simulink model "VCU_CS75_9_30"  (R2014a)
settings: Solver=FixedStepDiscrete  StartTime=0.0  StopTime=25  FixedStep=0.0005  RelTol=1e-3
undefined symbols (not defined in the file or in its folder): APAStatus_2D4, ecucoder_acal, I_SW01_L, LDW, ST_comd, TX2D4
libraries: simulink x881, ec5744lib x37
(part 8 of 30)

== system VCU_CS75_9_30/长安CS75底盘程序，20ms一次/BSW_Input/DBC转化的messages（存底）/ReceiveMessages4/EPB_256 ==
  input : Inport
  Demux : Demux  Outputs=8
  EPB_Checksum_Ad : Sum
  EPB_Checksum_Convert : DataTypeConversion  OutDataTypeStr=uint32
  EPB_Checksum_F : Gain
  EPB_Checksum_L : simulink/Logic and Bit Operations/Bitwise Operator  logicop=AND  UseBitMask=on  BitMask=255  BitMaskRealWorld=Stored Integer
  EPB_Checksum_O : Constant  Value=0  OutDataTypeStr=single
  EPB_Checksum_S : ArithShift
  EPB_Checksum_Sub : Subsystem
  EPB_Checksum_sat : Saturate  UpperLimit=255  LowerLimit=0
  EPB_Checksumcv : DataTypeConversion
  EPB_FailStatus_Ad : Sum
  EPB_FailStatus_Convert : DataTypeConversion  OutDataTypeStr=uint32
  EPB_FailStatus_F : Gain
  EPB_FailStatus_L : simulink/Logic and Bit Operations/Bitwise Operator  logicop=AND  UseBitMask=on  BitMask=192  BitMaskRealWorld=Stored Integer
  EPB_FailStatus_O : Constant  Value=0  OutDataTypeStr=single
  EPB_FailStatus_S : ArithShift  BitShiftNumber=6
  EPB_FailStatus_Sub : Subsystem
  EPB_FailStatus_sat : Saturate  UpperLimit=3  LowerLimit=0
  EPB_FailStatuscv : DataTypeConversion
  EPB_FailureLamp_Ad : Sum
  EPB_FailureLamp_Convert : DataTypeConversion  OutDataTypeStr=uint32
  EPB_FailureLamp_F : Gain
  EPB_FailureLamp_L : simulink/Logic and Bit Operations/Bitwise Operator  logicop=AND  UseBitMask=on  BitMask=48  BitMaskRealWorld=Stored Integer
  EPB_FailureLamp_O : Constant  Value=0  OutDataTypeStr=single
  EPB_FailureLamp_S : ArithShift  BitShiftNumber=4
  EPB_FailureLamp_Sub : Subsystem
  EPB_FailureLamp_sat : Saturate  UpperLimit=3  LowerLimit=0
  EPB_FailureLampcv : DataTypeConversion
  EPB_FunctionLamp_Ad : Sum
  EPB_FunctionLamp_Convert : DataTypeConversion  OutDataTypeStr=uint32
  EPB_FunctionLamp_F : Gain
  EPB_FunctionLamp_L : simulink/Logic and Bit Operations/Bitwise Operator  logicop=AND  UseBitMask=on  BitMask=12  BitMaskRealWorld=Stored Integer
  EPB_FunctionLamp_O : Constant  Value=0  OutDataTypeStr=single
  EPB_FunctionLamp_S : ArithShift  BitShiftNumber=2
  EPB_FunctionLamp_Sub : Subsystem
  EPB_FunctionLamp_sat : Saturate  UpperLimit=3  LowerLimit=0
  EPB_FunctionLampcv : DataTypeConversion
  EPB_RollingCounter_id256_Ad : Sum
  EPB_RollingCounter_id256_Convert : DataTypeConversion  OutDataTypeStr=uint32
  EPB_RollingCounter_id256_F : Gain
  EPB_RollingCounter_id256_L : simulink/Logic and Bit Operations/Bitwise Operator  logicop=AND  UseBitMask=on  BitMask=15  BitMaskRealWorld=Stored Integer
  EPB_RollingCounter_id256_O : Constant  Value=0  OutDataTypeStr=single
  EPB_RollingCounter_id256_S : ArithShift
  EPB_RollingCounter_id256_Sub : Subsystem
  EPB_RollingCounter_id256_sat : Saturate  UpperLimit=15  LowerLimit=0
  EPB_RollingCounter_id256cv : DataTypeConversion
  EPB_Status_Ad : Sum
  EPB_Status_Convert : DataTypeConversion  OutDataTypeStr=uint32
  EPB_Status_F : Gain
  EPB_Status_L : simulink/Logic and Bit Operations/Bitwise Operator  logicop=AND  UseBitMask=on  BitMask=192  BitMaskRealWorld=Stored Integer
  EPB_Status_O : Constant  Value=0  OutDataTypeStr=single
  EPB_Status_S : ArithShift  BitShiftNumber=6
  EPB_Status_Sub : Subsystem
  EPB_Status_sat : Saturate  UpperLimit=3  LowerLimit=0
  EPB_Statuscv : DataTypeConversion
  EPB_FailStatus_Out : Outport
  EPB_Status_Out : Outport  Port=2
  EPB_FunctionLamp_Out : Outport  Port=3
  EPB_FailureLamp_Out : Outport  Port=4
  EPB_RollingCounter_id256_Out : Outport  Port=5
  EPB_Checksum_Out : Outport  Port=6
  wires:
  EPB_FailStatus_F/1 -> EPB_FailStatus_Ad/1
  EPB_FailStatus_O/1 -> EPB_FailStatus_Ad/2
  EPB_FailStatus_Ad/1 -> EPB_FailStatus_sat/1
  EPB_FailStatus_sat/1 -> EPB_FailStatus_Out/1
  Demux/1 -> EPB_FailStatus_Sub/1(In1)
  EPB_FailStatus_Sub/1(Out1) -> EPB_FailStatus_Convert/1
  EPB_FailStatus_Convert/1 -> EPB_FailStatus_L/1
  EPB_FailStatus_L/1 -> EPB_FailStatus_S/1
  EPB_FailStatus_S/1 -> EPB_FailStatuscv/1
  EPB_FailStatuscv/1 -> EPB_FailStatus_F/1
  EPB_Status_F/1 -> EPB_Status_Ad/1
  EPB_Status_O/1 -> EPB_Status_Ad/2
  EPB_Status_Ad/1 -> EPB_Status_sat/1
  EPB_Status_sat/1 -> EPB_Status_Out/1
  Demux/3 -> EPB_Status_Sub/1(In1)
  EPB_Status_Sub/1(Out1) -> EPB_Status_Convert/1
  EPB_Status_Convert/1 -> EPB_Status_L/1
  EPB_Status_L/1 -> EPB_Status_S/1
  EPB_Status_S/1 -> EPB_Statuscv/1
  EPB_Statuscv/1 -> EPB_Status_F/1
  EPB_FunctionLamp_F/1 -> EPB_FunctionLamp_Ad/1
  EPB_FunctionLamp_O/1 -> EPB_FunctionLamp_Ad/2
  EPB_FunctionLamp_Ad/1 -> EPB_FunctionLamp_sat/1
  EPB_FunctionLamp_sat/1 -> EPB_FunctionLamp_Out/1
  Demux/6 -> EPB_FunctionLamp_Sub/1(In1), EPB_FailureLamp_Sub/1(In1)
  EPB_FunctionLamp_Sub/1(Out1) -> EPB_FunctionLamp_Convert/1
  EPB_FunctionLamp_Convert/1 -> EPB_FunctionLamp_L/1
  EPB_FunctionLamp_L/1 -> EPB_FunctionLamp_S/1
  EPB_FunctionLamp_S/1 -> EPB_FunctionLampcv/1
  EPB_FunctionLampcv/1 -> EPB_FunctionLamp_F/1
  EPB_FailureLamp_F/1 -> EPB_FailureLamp_Ad/1
  EPB_FailureLamp_O/1 -> EPB_FailureLamp_Ad/2
  EPB_FailureLamp_Ad/1 -> EPB_FailureLamp_sat/1
  EPB_FailureLamp_sat/1 -> EPB_FailureLamp_Out/1
  EPB_FailureLamp_Sub/1(Out1) -> EPB_FailureLamp_Convert/1
  EPB_FailureLamp_Convert/1 -> EPB_FailureLamp_L/1
  EPB_FailureLamp_L/1 -> EPB_FailureLamp_S/1
  EPB_FailureLamp_S/1 -> EPB_FailureLampcv/1
  EPB_FailureLampcv/1 -> EPB_FailureLamp_F/1
  EPB_RollingCounter_id256_F/1 -> EPB_RollingCounter_id256_Ad/1
  EPB_RollingCounter_id256_O/1 -> EPB_RollingCounter_id256_Ad/2
  EPB_RollingCounter_id256_Ad/1 -> EPB_RollingCounter_id256_sat/1
  EPB_RollingCounter_id256_sat/1 -> EPB_RollingCounter_id256_Out/1
  Demux/7 -> EPB_RollingCounter_id256_Sub/1(In1)
  EPB_RollingCounter_id256_Sub/1(Out1) -> EPB_RollingCounter_id256_Convert/1
  EPB_RollingCounter_id256_Convert/1 -> EPB_RollingCounter_id256_L/1
  EPB_RollingCounter_id256_L/1 -> EPB_RollingCounter_id256_S/1
  EPB_RollingCounter_id256_S/1 -> EPB_RollingCounter_id256cv/1
  EPB_RollingCounter_id256cv/1 -> EPB_RollingCounter_id256_F/1
  EPB_Checksum_F/1 -> EPB_Checksum_Ad/1
  EPB_Checksum_O/1 -> EPB_Checksum_Ad/2
  EPB_Checksum_Ad/1 -> EPB_Checksum_sat/1
  EPB_Checksum_sat/1 -> EPB_Checksum_Out/1
  Demux/8 -> EPB_Checksum_Sub/1(In1)
  EPB_Checksum_Sub/1(Out1) -> EPB_Checksum_Convert/1
  EPB_Checksum_Convert/1 -> EPB_Checksum_L/1
  EPB_Checksum_L/1 -> EPB_Checksum_S/1
  EPB_Checksum_S/1 -> EPB_Checksumcv/1
  EPB_Checksumcv/1 -> EPB_Checksum_F/1
  input/1 -> Demux/1

== system VCU_CS75_9_30/长安CS75底盘程序，20ms一次/BSW_Input/DBC转化的messages（存底）/ReceiveMessages5/EPS_20A ==
  input : Inport
  Demux : Demux  Outputs=8
  EPS_APA_AbortFeedback_Ad : Sum
  EPS_APA_AbortFeedback_Convert : DataTypeConversion  OutDataTypeStr=uint32
  EPS_APA_AbortFeedback_F : Gain
  EPS_APA_AbortFeedback_L : simulink/Logic and Bit Operations/Bitwise Operator  logicop=AND  UseBitMask=on  BitMask=112  BitMaskRealWorld=Stored Integer
  EPS_APA_AbortFeedback_O : Constant  Value=0  OutDataTypeStr=single
  EPS_APA_AbortFeedback_S : ArithShift  BitShiftNumber=4
  EPS_APA_AbortFeedback_Sub : Subsystem
  EPS_APA_AbortFeedback_sat : Saturate  UpperLimit=7  LowerLimit=0
  EPS_APA_AbortFeedbackcv : DataTypeConversion
  EPS_APA_ControlFeedback_Ad : Sum
  EPS_APA_ControlFeedback_Convert : DataTypeConversion  OutDataTypeStr=uint32
  EPS_APA_ControlFeedback_F : Gain
  EPS_APA_ControlFeedback_L : simulink/Logic and Bit Operations/Bitwise Operator  logicop=AND  UseBitMask=on  BitMask=64  BitMaskRealWorld=Stored Integer
  EPS_APA_ControlFeedback_O : Constant  Value=0  OutDataTypeStr=single
  EPS_APA_ControlFeedback_S : ArithShift  BitShiftNumber=6
  EPS_APA_ControlFeedback_Sub : Subsystem
  EPS_APA_ControlFeedback_sat : Saturate  UpperLimit=1  LowerLimit=0
  EPS_APA_ControlFeedbackcv : DataTypeConversion
  EPS_APA_EpasFailed_Ad : Sum
  EPS_APA_EpasFailed_Convert : DataTypeConversion  OutDataTypeStr=uint32
  EPS_APA_EpasFailed_F : Gain
  EPS_APA_EpasFailed_L : simulink/Logic and Bit Operations/Bitwise Operator  logicop=AND  UseBitMask=on  BitMask=2  BitMaskRealWorld=Stored Integer
  EPS_APA_EpasFailed_O : Constant  Value=0  OutDataTypeStr=single
  EPS_APA_EpasFailed_S : ArithShift  BitShiftNumber=1
  EPS_APA_EpasFailed_Sub : Subsystem
  EPS_APA_EpasFailed_sat : Saturate  UpperLimit=1  LowerLimit=0
  EPS_APA_EpasFailedcv : DataTypeConversion
  EPS_Checksum_Ad : Sum
  EPS_Checksum_Convert : DataTypeConversion  OutDataTypeStr=uint32
  EPS_Checksum_F : Gain
  EPS_Checksum_L : simulink/Logic and Bit Operations/Bitwise Operator  logicop=AND  UseBitMask=on  BitMask=255  BitMaskRealWorld=Stored Integer
  EPS_Checksum_O : Constant  Value=0  OutDataTypeStr=single
  EPS_Checksum_S : ArithShift
  EPS_Checksum_Sub : Subsystem
  EPS_Checksum_sat : Saturate  UpperLimit=255  LowerLimit=0
  EPS_Checksumcv : DataTypeConversion
  EPS_ConcussAvailabilityStatus_Ad : Sum
  EPS_ConcussAvailabilityStatus_Convert : DataTypeConversion  OutDataTypeStr=uint32
  EPS_ConcussAvailabilityStatus_F : Gain
  EPS_ConcussAvailabilityStatus_L : simulink/Logic and Bit Operations/Bitwise Operator  logicop=AND  UseBitMask=on  BitMask=48  BitMaskRealWorld=Stored Integer
  EPS_ConcussAvailabilityStatus_O : Constant  Value=0  OutDataTypeStr=single
  EPS_ConcussAvailabilityStatus_S : ArithShift  BitShiftNumber=4
  EPS_ConcussAvailabilityStatus_Sub : Subsystem
  EPS_ConcussAvailabilityStatus_sat : Saturate  UpperLimit=3  LowerLimit=0
  EPS_ConcussAvailabilityStatuscv : DataTypeConversion
  EPS_EPSFailed_Ad : Sum
  EPS_EPSFailed_Convert : DataTypeConversion  OutDataTypeStr=uint32
  EPS_EPSFailed_F : Gain
  EPS_EPSFailed_L : simulink/Logic and Bit Operations/Bitwise Operator  logicop=AND  UseBitMask=on  BitMask=128  BitMaskRealWorld=Stored Integer
  EPS_EPSFailed_O : Constant  Value=0  OutDataTypeStr=single
  EPS_EPSFailed_S : ArithShift  BitShiftNumber=7
  EPS_EPSFailed_Sub : Subsystem
  EPS_EPSFailed_sat : Saturate  UpperLimit=1  LowerLimit=0
  EPS_EPSFailedcv : DataTypeConversion
  EPS_RollingCounter_Ad : Sum
  EPS_RollingCounter_Convert : DataTypeConversion  OutDataTypeStr=uint32
  EPS_RollingCounter_F : Gain
  EPS_RollingCounter_L : simulink/Logic and Bit Operations/Bitwise Operator  logicop=AND  UseBitMask=on  BitMask=15  BitMaskRealWorld=Stored Integer
  EPS_RollingCounter_O : Constant  Value=0  OutDataTypeStr=single
  EPS_RollingCounter_S : ArithShift
  EPS_RollingCounter_Sub : Subsystem
  EPS_RollingCounter_sat : Saturate  UpperLimit=15  LowerLimit=0
  EPS_RollingCountercv : DataTypeConversion
  EPS_SteeringTorque_Ad : Sum
  EPS_SteeringTorque_Convert : DataTypeConversion  OutDataTypeStr=uint32
  EPS_SteeringTorque_F : Gain  Gain=0.1794
  EPS_SteeringTorque_L : simulink/Logic and Bit Operations/Bitwise Operator  logicop=AND  UseBitMask=on  BitMask=4080  BitMaskRealWorld=Stored Integer
  EPS_SteeringTorque_O : Constant  Value=-22.78  OutDataTypeStr=single
  EPS_SteeringTorque_S : ArithShift  BitShiftNumber=4
  EPS_SteeringTorque_Sub : Subsystem
  EPS_SteeringTorque_sat : Saturate  UpperLimit=22.78  LowerLimit=-22.78
  EPS_SteeringTorquecv : DataTypeConversion
  EPS_SteeringTorqueinput3_Ad : Sum
  EPS_SteeringTorqueinput3_C : Constant  Value=256
  EPS_SteeringTorqueinput3_P : Product
  EPS_TorqueSensorStatus_Ad : Sum
  EPS_TorqueSensorStatus_Convert : DataTypeConversion  OutDataTypeStr=uint32
  EPS_TorqueSensorStatus_F : Gain
  EPS_TorqueSensorStatus_L : simulink/Logic and Bit Operations/Bitwise Operator  logicop=AND  UseBitMask=on  BitMask=2  BitMaskRealWorld=Stored Integer
  EPS_TorqueSensorStatus_O : Constant  Value=0  OutDataTypeStr=single
  EPS_TorqueSensorStatus_S : ArithShift  BitShiftNumber=1
  EPS_TorqueSensorStatus_Sub : Subsystem
  EPS_TorqueSensorStatus_sat : Saturate  UpperLimit=1  LowerLimit=0
  EPS_TorqueSensorStatuscv : DataTypeConversion
  EPS_EPSFailed_Out : Outport
  EPS_APA_EpasFailed_Out : Outport  Port=2
  EPS_APA_AbortFeedback_Out : Outport  Port=3
  EPS_SteeringTorque_Out : Outport  Port=4
  EPS_TorqueSensorStatus_Out : Outport  Port=5
  EPS_APA_ControlFeedback_Out : Outport  Port=6
  EPS_RollingCounter_Out : Outport  Port=7
  EPS_ConcussAvailabilityStatus_Out : Outport  Port=8
  EPS_Checksum_Out : Outport  Port=9
  wires:
  EPS_EPSFailed_F/1 -> EPS_EPSFailed_Ad/1
  EPS_EPSFailed_O/1 -> EPS_EPSFailed_Ad/2
  EPS_EPSFailed_Ad/1 -> EPS_EPSFailed_sat/1
  EPS_EPSFailed_sat/1 -> EPS_EPSFailed_Out/1
  Demux/1 -> EPS_EPSFailed_Sub/1(In1)
  EPS_EPSFailed_Sub/1(Out1) -> EPS_EPSFailed_Convert/1
  EPS_EPSFailed_Convert/1 -> EPS_EPSFailed_L/1
  EPS_EPSFailed_L/1 -> EPS_EPSFailed_S/1
  EPS_EPSFailed_S/1 -> EPS_EPSFailedcv/1
  EPS_EPSFailedcv/1 -> EPS_EPSFailed_F/1
  EPS_APA_EpasFailed_F/1 -> EPS_APA_EpasFailed_Ad/1
  EPS_APA_EpasFailed_O/1 -> EPS_APA_EpasFailed_Ad/2
  EPS_APA_EpasFailed_Ad/1 -> EPS_APA_EpasFailed_sat/1
  EPS_APA_EpasFailed_sat/1 -> EPS_APA_EpasFailed_Out/1
  Demux/2 -> EPS_APA_EpasFailed_Sub/1(In1), EPS_APA_AbortFeedback_Sub/1(In1)
  EPS_APA_EpasFailed_Sub/1(Out1) -> EPS_APA_EpasFailed_Convert/1
  EPS_APA_EpasFailed_Convert/1 -> EPS_APA_EpasFailed_L/1
  EPS_APA_EpasFailed_L/1 -> EPS_APA_EpasFailed_S/1
  EPS_APA_EpasFailed_S/1 -> EPS_APA_EpasFailedcv/1
  EPS_APA_EpasFailedcv/1 -> EPS_APA_EpasFailed_F/1
  EPS_APA_AbortFeedback_F/1 -> EPS_APA_AbortFeedback_Ad/1
  EPS_APA_AbortFeedback_O/1 -> EPS_APA_AbortFeedback_Ad/2
  EPS_APA_AbortFeedback_Ad/1 -> EPS_APA_AbortFeedback_sat/1
  EPS_APA_AbortFeedback_sat/1 -> EPS_APA_AbortFeedback_Out/1
  EPS_APA_AbortFeedback_Sub/1(Out1) -> EPS_APA_AbortFeedback_Convert/1
  EPS_APA_AbortFeedback_Convert/1 -> EPS_APA_AbortFeedback_L/1
  EPS_APA_AbortFeedback_L/1 -> EPS_APA_AbortFeedback_S/1
  EPS_APA_AbortFeedback_S/1 -> EPS_APA_AbortFeedbackcv/1
  EPS_APA_AbortFeedbackcv/1 -> EPS_APA_AbortFeedback_F/1
  EPS_SteeringTorque_F/1 -> EPS_SteeringTorque_Ad/1
  EPS_SteeringTorque_O/1 -> EPS_SteeringTorque_Ad/2
  EPS_SteeringTorque_Ad/1 -> EPS_SteeringTorque_sat/1
  EPS_SteeringTorque_sat/1 -> EPS_SteeringTorque_Out/1
  Demux/3 -> EPS_SteeringTorqueinput3_P/1
  EPS_SteeringTorqueinput3_C/1 -> EPS_SteeringTorqueinput3_P/2
  EPS_SteeringTorqueinput3_P/1 -> EPS_SteeringTorqueinput3_Ad/1
  Demux/4 -> EPS_SteeringTorqueinput3_Ad/2
  EPS_SteeringTorqueinput3_Ad/1 -> EPS_SteeringTorque_Sub/1(In1)
  EPS_SteeringTorque_Sub/1(Out1) -> EPS_SteeringTorque_Convert/1
  EPS_SteeringTorque_Convert/1 -> EPS_SteeringTorque_L/1
  EPS_SteeringTorque_L/1 -> EPS_SteeringTorque_S/1
  EPS_SteeringTorque_S/1 -> EPS_SteeringTorquecv/1
  EPS_SteeringTorquecv/1 -> EPS_SteeringTorque_F/1
  EPS_TorqueSensorStatus_F/1 -> EPS_TorqueSensorStatus_Ad/1
  EPS_TorqueSensorStatus_O/1 -> EPS_TorqueSensorStatus_Ad/2
  EPS_TorqueSensorStatus_Ad/1 -> EPS_TorqueSensorStatus_sat/1
  EPS_TorqueSensorStatus_sat/1 -> EPS_TorqueSensorStatus_Out/1
  Demux/5 -> EPS_TorqueSensorStatus_Sub/1(In1)
  EPS_TorqueSensorStatus_Sub/1(Out1) -> EPS_TorqueSensorStatus_Convert/1
  EPS_TorqueSensorStatus_Convert/1 -> EPS_TorqueSensorStatus_L/1
  EPS_TorqueSensorStatus_L/1 -> EPS_TorqueSensorStatus_S/1
  EPS_TorqueSensorStatus_S/1 -> EPS_TorqueSensorStatuscv/1
  EPS_TorqueSensorStatuscv/1 -> EPS_TorqueSensorStatus_F/1
  EPS_APA_ControlFeedback_F/1 -> EPS_APA_ControlFeedback_Ad/1
  EPS_APA_ControlFeedback_O/1 -> EPS_APA_ControlFeedback_Ad/2
  EPS_APA_ControlFeedback_Ad/1 -> EPS_APA_ControlFeedback_sat/1
  EPS_APA_ControlFeedback_sat/1 -> EPS_APA_ControlFeedback_Out/1
  Demux/6 -> EPS_APA_ControlFeedback_Sub/1(In1)
  EPS_APA_ControlFeedback_Sub/1(Out1) -> EPS_APA_ControlFeedback_Convert/1
  EPS_APA_ControlFeedback_Convert/1 -> EPS_APA_ControlFeedback_L/1
  EPS_APA_ControlFeedback_L/1 -> EPS_APA_ControlFeedback_S/1
  EPS_APA_ControlFeedback_S/1 -> EPS_APA_ControlFeedbackcv/1
  EPS_APA_ControlFeedbackcv/1 -> EPS_APA_ControlFeedback_F/1
  EPS_RollingCounter_F/1 -> EPS_RollingCounter_Ad/1
  EPS_RollingCounter_O/1 -> EPS_RollingCounter_Ad/2
  EPS_RollingCounter_Ad/1 -> EPS_RollingCounter_sat/1
  EPS_RollingCounter_sat/1 -> EPS_RollingCounter_Out/1
  Demux/7 -> EPS_RollingCounter_Sub/1(In1), EPS_ConcussAvailabilityStatus_Sub/1(In1)
  EPS_RollingCounter_Sub/1(Out1) -> EPS_RollingCounter_Convert/1
  EPS_RollingCounter_Convert/1 -> EPS_RollingCounter_L/1
  EPS_RollingCounter_L/1 -> EPS_RollingCounter_S/1
  EPS_RollingCounter_S/1 -> EPS_RollingCountercv/1
  EPS_RollingCountercv/1 -> EPS_RollingCounter_F/1
  EPS_ConcussAvailabilityStatus_F/1 -> EPS_ConcussAvailabilityStatus_Ad/1
  EPS_ConcussAvailabilityStatus_O/1 -> EPS_ConcussAvailabilityStatus_Ad/2
  EPS_ConcussAvailabilityStatus_Ad/1 -> EPS_ConcussAvailabilityStatus_sat/1
  EPS_ConcussAvailabilityStatus_sat/1 -> EPS_ConcussAvailabilityStatus_Out/1
  EPS_ConcussAvailabilityStatus_Sub/1(Out1) -> EPS_ConcussAvailabilityStatus_Convert/1
  EPS_ConcussAvailabilityStatus_Convert/1 -> EPS_ConcussAvailabilityStatus_L/1
  EPS_ConcussAvailabilityStatus_L/1 -> EPS_ConcussAvailabilityStatus_S/1
  EPS_ConcussAvailabilityStatus_S/1 -> EPS_ConcussAvailabilityStatuscv/1
  EPS_ConcussAvailabilityStatuscv/1 -> EPS_ConcussAvailabilityStatus_F/1
  EPS_Checksum_F/1 -> EPS_Checksum_Ad/1
  EPS_Checksum_O/1 -> EPS_Checksum_Ad/2
  EPS_Checksum_Ad/1 -> EPS_Checksum_sat/1
  EPS_Checksum_sat/1 -> EPS_Checksum_Out/1
  Demux/8 -> EPS_Checksum_Sub/1(In1)
  EPS_Checksum_Sub/1(Out1) -> EPS_Checksum_Convert/1
  EPS_Checksum_Convert/1 -> EPS_Checksum_L/1
  EPS_Checksum_L/1 -> EPS_Checksum_S/1
  EPS_Checksum_S/1 -> EPS_Checksumcv/1
  EPS_Checksumcv/1 -> EPS_Checksum_F/1
  input/1 -> Demux/1

== system VCU_CS75_9_30/长安CS75底盘程序，20ms一次/BSW_Input/DBC转化的messages（存底）/ReceiveMessages6/EPS_21A ==
  input : Inport
  CRC_Ad : Sum
  CRC_Convert : DataTypeConversion  OutDataTypeStr=uint32
  CRC_F : Gain
  CRC_L : simulink/Logic and Bit Operations/Bitwise Operator  logicop=AND  UseBitMask=on  BitMask=255  BitMaskRealWorld=Stored Integer
  CRC_O : Constant  Value=0  OutDataTypeStr=single
  CRC_S : ArithShift
  CRC_Sub : Subsystem
  CRC_sat : Saturate  UpperLimit=0  LowerLimit=0
  CRCcv : DataTypeConversion
  Demux : Demux  Outputs=8
  EPS_AvailabilityStatus_Ad : Sum
  EPS_AvailabilityStatus_Convert : DataTypeConversion  OutDataTypeStr=uint32
  EPS_AvailabilityStatus_F : Gain
  EPS_AvailabilityStatus_L : simulink/Logic and Bit Operations/Bitwise Operator  logicop=AND  UseBitMask=on  BitMask=28  BitMaskRealWorld=Stored Integer
  EPS_AvailabilityStatus_O : Constant  Value=0  OutDataTypeStr=single
  EPS_AvailabilityStatus_S : ArithShift  BitShiftNumber=2
  EPS_AvailabilityStatus_Sub : Subsystem
  EPS_AvailabilityStatus_sat : Saturate  UpperLimit=7  LowerLimit=0
  EPS_AvailabilityStatuscv : DataTypeConversion
  EPS_IACC_abortReson_Ad : Sum
  EPS_IACC_abortReson_Convert : DataTypeConversion  OutDataTypeStr=uint32
  EPS_IACC_abortReson_F : Gain
  EPS_IACC_abortReson_L : simulink/Logic and Bit Operations/Bitwise Operator  logicop=AND  UseBitMask=on  BitMask=112  BitMaskRealWorld=Stored Integer
  EPS_IACC_abortReson_O : Constant  Value=0  OutDataTypeStr=single
  EPS_IACC_abortReson_S : ArithShift  BitShiftNumber=4
  EPS_IACC_abortReson_Sub : Subsystem
  EPS_IACC_abortReson_sat : Saturate  UpperLimit=7  LowerLimit=0
  EPS_IACC_abortResoncv : DataTypeConversion
  EPS_MeasTsionBatTorquevalid_Ad : Sum
  EPS_MeasTsionBatTorquevalid_Convert : DataTypeConversion  OutDataTypeStr=uint32
  EPS_MeasTsionBatTorquevalid_F : Gain
  EPS_MeasTsionBatTorquevalid_L : simulink/Logic and Bit Operations/Bitwise Operator  logicop=AND  UseBitMask=on  BitMask=64  BitMaskRealWorld=Stored Integer
  EPS_MeasTsionBatTorquevalid_O : Constant  Value=0  OutDataTypeStr=single
  EPS_MeasTsionBatTorquevalid_S : ArithShift  BitShiftNumber=6
  EPS_MeasTsionBatTorquevalid_Sub : Subsystem
  EPS_MeasTsionBatTorquevalid_sat : Saturate  UpperLimit=1  LowerLimit=0
  EPS_MeasTsionBatTorquevalidcv : DataTypeConversion
  EPS_MeasuredTosionBatTorque_Ad : Sum
  EPS_MeasuredTosionBatTorque_Convert : DataTypeConversion  OutDataTypeStr=uint32
  EPS_MeasuredTosionBatTorque_F : Gain  Gain=0.01
  EPS_MeasuredTosionBatTorque_L : simulink/Logic and Bit Operations/Bitwise Operator  logicop=AND  UseBitMask=on  BitMask=65504  BitMaskRealWorld=Stored Integer
  EPS_MeasuredTosionBatTorque_O : Constant  Value=-10.23  OutDataTypeStr=single
  EPS_MeasuredTosionBatTorque_S : ArithShift  BitShiftNumber=5
  EPS_MeasuredTosionBatTorque_Sub : Subsystem
  EPS_MeasuredTosionBatTorque_sat : Saturate  UpperLimit=10.23  LowerLimit=-10.23
  EPS_MeasuredTosionBatTorquecv : DataTypeConversion
  EPS_MeasuredTosionBatTorqueinput1_Ad : Sum
  EPS_MeasuredTosionBatTorqueinput1_C : Constant  Value=256
  EPS_MeasuredTosionBatTorqueinput1_P : Product
  Rollingcounter_Ad : Sum
  Rollingcounter_Convert : DataTypeConversion  OutDataTypeStr=uint32
  Rollingcounter_F : Gain
  Rollingcounter_L : simulink/Logic and Bit Operations/Bitwise Operator  logicop=AND  UseBitMask=on  BitMask=15  BitMaskRealWorld=Stored Integer
  Rollingcounter_O : Constant  Value=0  OutDataTypeStr=single
  Rollingcounter_S : ArithShift
  Rollingcounter_Sub : Subsystem
  Rollingcounter_sat : Saturate  UpperLimit=15  LowerLimit=0
  Rollingcountercv : DataTypeConversion
  EPS_MeasuredTosionBatTorque_Out : Outport
  EPS_AvailabilityStatus_Out : Outport  Port=2
  EPS_MeasTsionBatTorquevalid_Out : Outport  Port=3
  EPS_IACC_abortReson_Out : Outport  Port=4
  Rollingcounter_Out : Outport  Port=5
  CRC_Out : Outport  Port=6
  wires:
  input/1 -> Demux/1
  CRCcv/1 -> CRC_F/1
  CRC_S/1 -> CRCcv/1
  CRC_L/1 -> CRC_S/1
  CRC_Convert/1 -> CRC_L/1
  CRC_Sub/1(Out1) -> CRC_Convert/1
  Demux/8 -> CRC_Sub/1(In1)
  CRC_sat/1 -> CRC_Out/1
  CRC_Ad/1 -> CRC_sat/1
  CRC_O/1 -> CRC_Ad/2
  CRC_F/1 -> CRC_Ad/1
  Rollingcountercv/1 -> Rollingcounter_F/1
  Rollingcounter_S/1 -> Rollingcountercv/1
  Rollingcounter_L/1 -> Rollingcounter_S/1
  Rollingcounter_Convert/1 -> Rollingcounter_L/1
  Rollingcounter_Sub/1(Out1) -> Rollingcounter_Convert/1
  Demux/7 -> Rollingcounter_Sub/1(In1)
  Rollingcounter_sat/1 -> Rollingcounter_Out/1
  Rollingcounter_Ad/1 -> Rollingcounter_sat/1
  Rollingcounter_O/1 -> Rollingcounter_Ad/2
  Rollingcounter_F/1 -> Rollingcounter_Ad/1
  EPS_IACC_abortResoncv/1 -> EPS_IACC_abortReson_F/1
  EPS_IACC_abortReson_S/1 -> EPS_IACC_abortResoncv/1
  EPS_IACC_abortReson_L/1 -> EPS_IACC_abortReson_S/1
  EPS_IACC_abortReson_Convert/1 -> EPS_IACC_abortReson_L/1
  EPS_IACC_abortReson_Sub/1(Out1) -> EPS_IACC_abortReson_Convert/1
  Demux/6 -> EPS_IACC_abortReson_Sub/1(In1)
  EPS_IACC_abortReson_sat/1 -> EPS_IACC_abortReson_Out/1
  EPS_IACC_abortReson_Ad/1 -> EPS_IACC_abortReson_sat/1
  EPS_IACC_abortReson_O/1 -> EPS_IACC_abortReson_Ad/2
  EPS_IACC_abortReson_F/1 -> EPS_IACC_abortReson_Ad/1
  EPS_MeasTsionBatTorquevalidcv/1 -> EPS_MeasTsionBatTorquevalid_F/1
  EPS_MeasTsionBatTorquevalid_S/1 -> EPS_MeasTsionBatTorquevalidcv/1
  EPS_MeasTsionBatTorquevalid_L/1 -> EPS_MeasTsionBatTorquevalid_S/1
  EPS_MeasTsionBatTorquevalid_Convert/1 -> EPS_MeasTsionBatTorquevalid_L/1
  EPS_MeasTsionBatTorquevalid_Sub/1(Out1) -> EPS_MeasTsionBatTorquevalid_Convert/1
  Demux/5 -> EPS_MeasTsionBatTorquevalid_Sub/1(In1)
  EPS_MeasTsionBatTorquevalid_sat/1 -> EPS_MeasTsionBatTorquevalid_Out/1
  EPS_MeasTsionBatTorquevalid_Ad/1 -> EPS_MeasTsionBatTorquevalid_sat/1
  EPS_MeasTsionBatTorquevalid_O/1 -> EPS_MeasTsionBatTorquevalid_Ad/2
  EPS_MeasTsionBatTorquevalid_F/1 -> EPS_MeasTsionBatTorquevalid_Ad/1
  EPS_AvailabilityStatuscv/1 -> EPS_AvailabilityStatus_F/1
  EPS_AvailabilityStatus_S/1 -> EPS_AvailabilityStatuscv/1
  EPS_AvailabilityStatus_L/1 -> EPS_AvailabilityStatus_S/1
  EPS_AvailabilityStatus_Convert/1 -> EPS_AvailabilityStatus_L/1
  EPS_AvailabilityStatus_Sub/1(Out1) -> EPS_AvailabilityStatus_Convert/1
  Demux/3 -> EPS_AvailabilityStatus_Sub/1(In1)
  EPS_AvailabilityStatus_sat/1 -> EPS_AvailabilityStatus_Out/1
  EPS_AvailabilityStatus_Ad/1 -> EPS_AvailabilityStatus_sat/1
  EPS_AvailabilityStatus_O/1 -> EPS_AvailabilityStatus_Ad/2
  EPS_AvailabilityStatus_F/1 -> EPS_AvailabilityStatus_Ad/1
  EPS_MeasuredTosionBatTorquecv/1 -> EPS_MeasuredTosionBatTorque_F/1
  EPS_MeasuredTosionBatTorque_S/1 -> EPS_MeasuredTosionBatTorquecv/1
  EPS_MeasuredTosionBatTorque_L/1 -> EPS_MeasuredTosionBatTorque_S/1
  EPS_MeasuredTosionBatTorque_Convert/1 -> EPS_MeasuredTosionBatTorque_L/1
  EPS_MeasuredTosionBatTorque_Sub/1(Out1) -> EPS_MeasuredTosionBatTorque_Convert/1
  EPS_MeasuredTosionBatTorqueinput1_Ad/1 -> EPS_MeasuredTosionBatTorque_Sub/1(In1)
  Demux/2 -> EPS_MeasuredTosionBatTorqueinput1_Ad/2
  EPS_MeasuredTosionBatTorqueinput1_P/1 -> EPS_MeasuredTosionBatTorqueinput1_Ad/1
  EPS_MeasuredTosionBatTorqueinput1_C/1 -> EPS_MeasuredTosionBatTorqueinput1_P/2
  Demux/1 -> EPS_MeasuredTosionBatTorqueinput1_P/1
  EPS_MeasuredTosionBatTorque_sat/1 -> EPS_MeasuredTosionBatTorque_Out/1
  EPS_MeasuredTosionBatTorque_Ad/1 -> EPS_MeasuredTosionBatTorque_sat/1
  EPS_MeasuredTosionBatTorque_O/1 -> EPS_MeasuredTosionBatTorque_Ad/2
  EPS_MeasuredTosionBatTorque_F/1 -> EPS_MeasuredTosionBatTorque_Ad/1

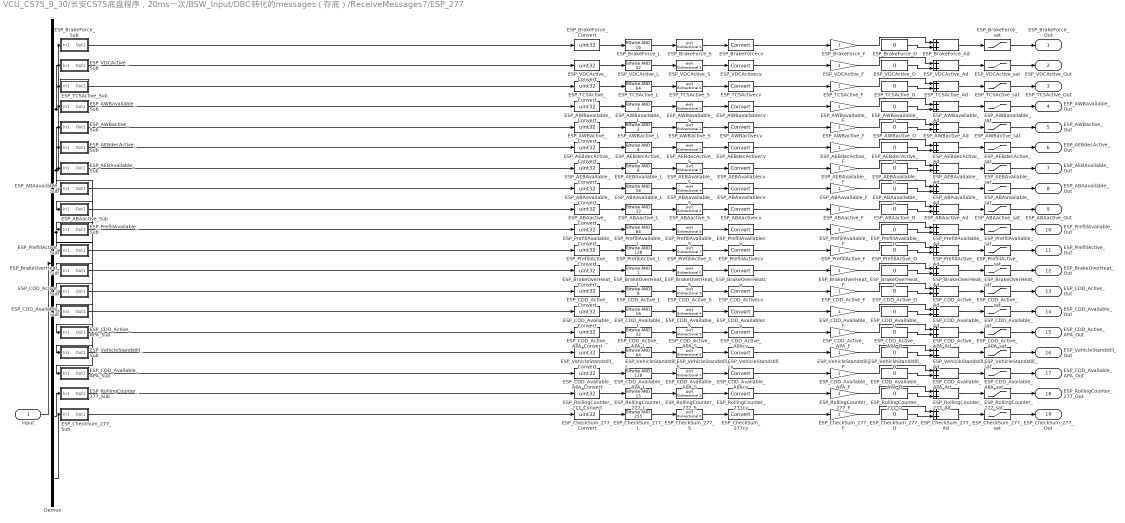
== system VCU_CS75_9_30/长安CS75底盘程序，20ms一次/BSW_Input/DBC转化的messages（存底）/ReceiveMessages7/ESP_277 ==
  input : Inport
  Demux : Demux  Outputs=8
  ESP_ABAactive_Ad : Sum
  ESP_ABAactive_Convert : DataTypeConversion  OutDataTypeStr=uint32
  ESP_ABAactive_F : Gain
  ESP_ABAactive_L : simulink/Logic and Bit Operations/Bitwise Operator  logicop=AND  UseBitMask=on  BitMask=32  BitMaskRealWorld=Stored Integer
  ESP_ABAactive_O : Constant  Value=0  OutDataTypeStr=single
  ESP_ABAactive_S : ArithShift  BitShiftNumber=5
  ESP_ABAactive_Sub : Subsystem
  ESP_ABAactive_sat : Saturate  UpperLimit=1  LowerLimit=0
  ESP_ABAactivecv : DataTypeConversion
  ESP_ABAavailable_Ad : Sum
  ESP_ABAavailable_Convert : DataTypeConversion  OutDataTypeStr=uint32
  ESP_ABAavailable_F : Gain
  ESP_ABAavailable_L : simulink/Logic and Bit Operations/Bitwise Operator  logicop=AND  UseBitMask=on  BitMask=16  BitMaskRealWorld=Stored Integer
  ESP_ABAavailable_O : Constant  Value=0  OutDataTypeStr=single
  ESP_ABAavailable_S : ArithShift  BitShiftNumber=4
  ESP_ABAavailable_Sub : Subsystem
  ESP_ABAavailable_sat : Saturate  UpperLimit=1  LowerLimit=0
  ESP_ABAavailablecv : DataTypeConversion
  ESP_AEBAvailable_Ad : Sum
  ESP_AEBAvailable_Convert : DataTypeConversion  OutDataTypeStr=uint32
  ESP_AEBAvailable_F : Gain
  ESP_AEBAvailable_L : simulink/Logic and Bit Operations/Bitwise Operator  logicop=AND  UseBitMask=on  BitMask=8  BitMaskRealWorld=Stored Integer
  ESP_AEBAvailable_O : Constant  Value=0  OutDataTypeStr=single
  ESP_AEBAvailable_S : ArithShift  BitShiftNumber=3
  ESP_AEBAvailable_Sub : Subsystem
  ESP_AEBAvailable_sat : Saturate  UpperLimit=1  LowerLimit=0
  ESP_AEBAvailablecv : DataTypeConversion
  ESP_AEBdecActive_Ad : Sum
  ESP_AEBdecActive_Convert : DataTypeConversion  OutDataTypeStr=uint32
  ESP_AEBdecActive_F : Gain
  ESP_AEBdecActive_L : simulink/Logic and Bit Operations/Bitwise Operator  logicop=AND  UseBitMask=on  BitMask=4  BitMaskRealWorld=Stored Integer
  ESP_AEBdecActive_O : Constant  Value=0  OutDataTypeStr=single
  ESP_AEBdecActive_S : ArithShift  BitShiftNumber=2
  ESP_AEBdecActive_Sub : Subsystem
  ESP_AEBdecActive_sat : Saturate  UpperLimit=1  LowerLimit=0
  ESP_AEBdecActivecv : DataTypeConversion
  ESP_AWBactive_Ad : Sum
  ESP_AWBactive_Convert : DataTypeConversion  OutDataTypeStr=uint32
  ESP_AWBactive_F : Gain
  ESP_AWBactive_L : simulink/Logic and Bit Operations/Bitwise Operator  logicop=AND  UseBitMask=on  BitMask=2  BitMaskRealWorld=Stored Integer
  ESP_AWBactive_O : Constant  Value=0  OutDataTypeStr=single
  ESP_AWBactive_S : ArithShift  BitShiftNumber=1
  ESP_AWBactive_Sub : Subsystem
  ESP_AWBactive_sat : Saturate  UpperLimit=1  LowerLimit=0
  ESP_AWBactivecv : DataTypeConversion
  ESP_AWBavailable_Ad : Sum
  ESP_AWBavailable_Convert : DataTypeConversion  OutDataTypeStr=uint32
  ESP_AWBavailable_F : Gain
  ESP_AWBavailable_L : simulink/Logic and Bit Operations/Bitwise Operator  logicop=AND  UseBitMask=on  BitMask=1  BitMaskRealWorld=Stored Integer
  ESP_AWBavailable_O : Constant  Value=0  OutDataTypeStr=single
  ESP_AWBavailable_S : ArithShift
  ESP_AWBavailable_Sub : Subsystem
  ESP_AWBavailable_sat : Saturate  UpperLimit=1  LowerLimit=0
  ESP_AWBavailablecv : DataTypeConversion
  ESP_BrakeForce_Ad : Sum
  ESP_BrakeForce_Convert : DataTypeConversion  OutDataTypeStr=uint32
  ESP_BrakeForce_F : Gain
  ESP_BrakeForce_L : simulink/Logic and Bit Operations/Bitwise Operator  logicop=AND  UseBitMask=on  BitMask=16  BitMaskRealWorld=Stored Integer
  ESP_BrakeForce_O : Constant  Value=0  OutDataTypeStr=single
  ESP_BrakeForce_S : ArithShift  BitShiftNumber=4
  ESP_BrakeForce_Sub : Subsystem
  ESP_BrakeForce_sat : Saturate  UpperLimit=1  LowerLimit=0
  ESP_BrakeForcecv : DataTypeConversion
  ESP_BrakeOverHeat_Ad : Sum
  ESP_BrakeOverHeat_Convert : DataTypeConversion  OutDataTypeStr=uint32
  ESP_BrakeOverHeat_F : Gain
  ESP_BrakeOverHeat_L : simulink/Logic and Bit Operations/Bitwise Operator  logicop=AND  UseBitMask=on  BitMask=1  BitMaskRealWorld=Stored Integer
  ESP_BrakeOverHeat_O : Constant  Value=0  OutDataTypeStr=single
  ESP_BrakeOverHeat_S : ArithShift
  ESP_BrakeOverHeat_Sub : Subsystem
  ESP_BrakeOverHeat_sat : Saturate  UpperLimit=1  LowerLimit=0
  ESP_BrakeOverHeatcv : DataTypeConversion
  ESP_CDD_Active_APA_Ad : Sum
  ESP_CDD_Active_APA_Convert : DataTypeConversion  OutDataTypeStr=uint32
  ESP_CDD_Active_APA_F : Gain
  ESP_CDD_Active_APA_L : simulink/Logic and Bit Operations/Bitwise Operator  logicop=AND  UseBitMask=on  BitMask=32  BitMaskRealWorld=Stored Integer
  ESP_CDD_Active_APA_O : Constant  Value=0  OutDataTypeStr=single
  ESP_CDD_Active_APA_S : ArithShift  BitShiftNumber=5
  ESP_CDD_Active_APA_Sub : Subsystem
  ESP_CDD_Active_APA_sat : Saturate  UpperLimit=0  LowerLimit=0
  ESP_CDD_Active_APAcv : DataTypeConversion
  ESP_CDD_Active_Ad : Sum
  ESP_CDD_Active_Convert : DataTypeConversion  OutDataTypeStr=uint32
  ESP_CDD_Active_F : Gain
  ESP_CDD_Active_L : simulink/Logic and Bit Operations/Bitwise Operator  logicop=AND  UseBitMask=on  BitMask=8  BitMaskRealWorld=Stored Integer
  ESP_CDD_Active_O : Constant  Value=0  OutDataTypeStr=single
  ESP_CDD_Active_S : ArithShift  BitShiftNumber=3
  ESP_CDD_Active_Sub : Subsystem
  ESP_CDD_Active_sat : Saturate  UpperLimit=1  LowerLimit=0
  ESP_CDD_Activecv : DataTypeConversion
  ESP_CDD_Available_APA_Ad : Sum
  ESP_CDD_Available_APA_Convert : DataTypeConversion  OutDataTypeStr=uint32
  ESP_CDD_Available_APA_F : Gain
  ESP_CDD_Available_APA_L : simulink/Logic and Bit Operations/Bitwise Operator  logicop=AND  UseBitMask=on  BitMask=128  BitMaskRealWorld=Stored Integer
  ESP_CDD_Available_APA_O : Constant  Value=0  OutDataTypeStr=single
  ESP_CDD_Available_APA_S : ArithShift  BitShiftNumber=7
  ESP_CDD_Available_APA_Sub : Subsystem
  ESP_CDD_Available_APA_sat : Saturate  UpperLimit=0  LowerLimit=0
  ESP_CDD_Available_APAcv : DataTypeConversion
  ESP_CDD_Available_Ad : Sum
  ESP_CDD_Available_Convert : DataTypeConversion  OutDataTypeStr=uint32
  ESP_CDD_Available_F : Gain
  ESP_CDD_Available_L : simulink/Logic and Bit Operations/Bitwise Operator  logicop=AND  UseBitMask=on  BitMask=16  BitMaskRealWorld=Stored Integer
  ESP_CDD_Available_O : Constant  Value=0  OutDataTypeStr=single
  ESP_CDD_Available_S : ArithShift  BitShiftNumber=4
  ESP_CDD_Available_Sub : Subsystem
  ESP_CDD_Available_sat : Saturate  UpperLimit=1  LowerLimit=0
  ESP_CDD_Availablecv : DataTypeConversion
  ESP_CheckSum_277_Ad : Sum
  ESP_CheckSum_277_Convert : DataTypeConversion  OutDataTypeStr=uint32
  ESP_CheckSum_277_F : Gain
  ESP_CheckSum_277_L : simulink/Logic and Bit Operations/Bitwise Operator  logicop=AND  UseBitMask=on  BitMask=255  BitMaskRealWorld=Stored Integer
  ESP_CheckSum_277_O : Constant  Value=0  OutDataTypeStr=single
  ESP_CheckSum_277_S : ArithShift
  ESP_CheckSum_277_Sub : Subsystem
  ESP_CheckSum_277_sat : Saturate  UpperLimit=255  LowerLimit=0
  ESP_CheckSum_277cv : DataTypeConversion
  ESP_PrefillActive_Ad : Sum
  ESP_PrefillActive_Convert : DataTypeConversion  OutDataTypeStr=uint32
  ESP_PrefillActive_F : Gain
  ESP_PrefillActive_L : simulink/Logic and Bit Operations/Bitwise Operator  logicop=AND  UseBitMask=on  BitMask=128  BitMaskRealWorld=Stored Integer
  ESP_PrefillActive_O : Constant  Value=0  OutDataTypeStr=single
  ESP_PrefillActive_S : ArithShift  BitShiftNumber=7
  ESP_PrefillActive_Sub : Subsystem
  ESP_PrefillActive_sat : Saturate  UpperLimit=1  LowerLimit=0
  ESP_PrefillActivecv : DataTypeConversion
  ESP_PrefillAvailable_Ad : Sum
  ESP_PrefillAvailable_Convert : DataTypeConversion  OutDataTypeStr=uint32
  ESP_PrefillAvailable_F : Gain
  ESP_PrefillAvailable_L : simulink/Logic and Bit Operations/Bitwise Operator  logicop=AND  UseBitMask=on  BitMask=64  BitMaskRealWorld=Stored Integer
  ESP_PrefillAvailable_O : Constant  Value=0  OutDataTypeStr=single
  ESP_PrefillAvailable_S : ArithShift  BitShiftNumber=6
  ESP_PrefillAvailable_Sub : Subsystem
  ESP_PrefillAvailable_sat : Saturate  UpperLimit=1  LowerLimit=0
  ESP_PrefillAvailablecv : DataTypeConversion
  ESP_RollingCounter_277_Ad : Sum
  ESP_RollingCounter_277_Convert : DataTypeConversion  OutDataTypeStr=uint32
  ESP_RollingCounter_277_F : Gain
  ESP_RollingCounter_277_L : simulink/Logic and Bit Operations/Bitwise Operator  logicop=AND  UseBitMask=on  BitMask=15  BitMaskRealWorld=Stored Integer
  ESP_RollingCounter_277_O : Constant  Value=0  OutDataTypeStr=single
  ESP_RollingCounter_277_S : ArithShift
  ESP_RollingCounter_277_Sub : Subsystem
  ESP_RollingCounter_277_sat : Saturate  UpperLimit=15  LowerLimit=0
  ESP_RollingCounter_277cv : DataTypeConversion
  ESP_TCSActive_Ad : Sum
  ESP_TCSActive_Convert : DataTypeConversion  OutDataTypeStr=uint32
  ESP_TCSActive_F : Gain
  ESP_TCSActive_L : simulink/Logic and Bit Operations/Bitwise Operator  logicop=AND  UseBitMask=on  BitMask=64  BitMaskRealWorld=Stored Integer
  ESP_TCSActive_O : Constant  Value=0  OutDataTypeStr=single
  ESP_TCSActive_S : ArithShift  BitShiftNumber=6
  ESP_TCSActive_Sub : Subsystem
  ESP_TCSActive_sat : Saturate  UpperLimit=1  LowerLimit=0
  ESP_TCSActivecv : DataTypeConversion
  ESP_VDCActive_Ad : Sum
  ESP_VDCActive_Convert : DataTypeConversion  OutDataTypeStr=uint32
  ESP_VDCActive_F : Gain
  ESP_VDCActive_L : simulink/Logic and Bit Operations/Bitwise Operator  logicop=AND  UseBitMask=on  BitMask=32  BitMaskRealWorld=Stored Integer
  ESP_VDCActive_O : Constant  Value=0  OutDataTypeStr=single
  ESP_VDCActive_S : ArithShift  BitShiftNumber=5
  ESP_VDCActive_Sub : Subsystem
  ESP_VDCActive_sat : Saturate  UpperLimit=1  LowerLimit=0
  ESP_VDCActivecv : DataTypeConversion
  ESP_VehicleStandstill_Ad : Sum
  ESP_VehicleStandstill_Convert : DataTypeConversion  OutDataTypeStr=uint32
  ESP_VehicleStandstill_F : Gain
  ESP_VehicleStandstill_L : simulink/Logic and Bit Operations/Bitwise Operator  logicop=AND  UseBitMask=on  BitMask=64  BitMaskRealWorld=Stored Integer
  ESP_VehicleStandstill_O : Constant  Value=0  OutDataTypeStr=single
  ESP_VehicleStandstill_S : ArithShift  BitShiftNumber=6
  ESP_VehicleStandstill_Sub : Subsystem
  ESP_VehicleStandstill_sat : Saturate  UpperLimit=1  LowerLimit=0
  ESP_VehicleStandstillcv : DataTypeConversion
  ESP_BrakeForce_Out : Outport
  ESP_VDCActive_Out : Outport  Port=2
  ESP_TCSActive_Out : Outport  Port=3
  ESP_AWBavailable_Out : Outport  Port=4
  ESP_AWBactive_Out : Outport  Port=5
  ESP_AEBdecActive_Out : Outport  Port=6
  ESP_AEBAvailable_Out : Outport  Port=7
  ESP_ABAavailable_Out : Outport  Port=8
  ESP_ABAactive_Out : Outport  Port=9
  ESP_PrefillAvailable_Out : Outport  Port=10
  ESP_PrefillActive_Out : Outport  Port=11
  ESP_BrakeOverHeat_Out : Outport  Port=12
  ESP_CDD_Active_Out : Outport  Port=13
  ESP_CDD_Available_Out : Outport  Port=14
  ESP_CDD_Active_APA_Out : Outport  Port=15
  ESP_VehicleStandstill_Out : Outport  Port=16
  ESP_CDD_Available_APA_Out : Outport  Port=17
  ESP_RollingCounter_277_Out : Outport  Port=18
  ESP_CheckSum_277_Out : Outport  Port=19
  wires:
  input/1 -> Demux/1
  ESP_CheckSum_277cv/1 -> ESP_CheckSum_277_F/1
  ESP_CheckSum_277_S/1 -> ESP_CheckSum_277cv/1
  ESP_CheckSum_277_L/1 -> ESP_CheckSum_277_S/1
  ESP_CheckSum_277_Convert/1 -> ESP_CheckSum_277_L/1
  ESP_CheckSum_277_Sub/1(Out1) -> ESP_CheckSum_277_Convert/1
  Demux/8 -> ESP_CheckSum_277_Sub/1(In1)
  ESP_CheckSum_277_sat/1 -> ESP_CheckSum_277_Out/1
  ESP_CheckSum_277_Ad/1 -> ESP_CheckSum_277_sat/1
  ESP_CheckSum_277_O/1 -> ESP_CheckSum_277_Ad/2
  ESP_CheckSum_277_F/1 -> ESP_CheckSum_277_Ad/1
  ESP_RollingCounter_277cv/1 -> ESP_RollingCounter_277_F/1
  ESP_RollingCounter_277_S/1 -> ESP_RollingCounter_277cv/1
  ESP_RollingCounter_277_L/1 -> ESP_RollingCounter_277_S/1
  ESP_RollingCounter_277_Convert/1 -> ESP_RollingCounter_277_L/1
  ESP_RollingCounter_277_Sub/1(Out1) -> ESP_RollingCounter_277_Convert/1
  Demux/7 -> ESP_RollingCounter_277_Sub/1(In1)
  ESP_RollingCounter_277_sat/1 -> ESP_RollingCounter_277_Out/1
  ESP_RollingCounter_277_Ad/1 -> ESP_RollingCounter_277_sat/1
  ESP_RollingCounter_277_O/1 -> ESP_RollingCounter_277_Ad/2
  ESP_RollingCounter_277_F/1 -> ESP_RollingCounter_277_Ad/1
  ESP_CDD_Available_APAcv/1 -> ESP_CDD_Available_APA_F/1
  ESP_CDD_Available_APA_S/1 -> ESP_CDD_Available_APAcv/1
  ESP_CDD_Available_APA_L/1 -> ESP_CDD_Available_APA_S/1
  ESP_CDD_Available_APA_Convert/1 -> ESP_CDD_Available_APA_L/1
  ESP_CDD_Available_APA_Sub/1(Out1) -> ESP_CDD_Available_APA_Convert/1
  ESP_CDD_Available_APA_sat/1 -> ESP_CDD_Available_APA_Out/1
  ESP_CDD_Available_APA_Ad/1 -> ESP_CDD_Available_APA_sat/1
  ESP_CDD_Available_APA_O/1 -> ESP_CDD_Available_APA_Ad/2
  ESP_CDD_Available_APA_F/1 -> ESP_CDD_Available_APA_Ad/1
  ESP_VehicleStandstillcv/1 -> ESP_VehicleStandstill_F/1
  ESP_VehicleStandstill_S/1 -> ESP_VehicleStandstillcv/1
  ESP_VehicleStandstill_L/1 -> ESP_VehicleStandstill_S/1
  ESP_VehicleStandstill_Convert/1 -> ESP_VehicleStandstill_L/1
  ESP_VehicleStandstill_Sub/1(Out1) -> ESP_VehicleStandstill_Convert/1
  ESP_VehicleStandstill_sat/1 -> ESP_VehicleStandstill_Out/1
  ESP_VehicleStandstill_Ad/1 -> ESP_VehicleStandstill_sat/1
  ESP_VehicleStandstill_O/1 -> ESP_VehicleStandstill_Ad/2
  ESP_VehicleStandstill_F/1 -> ESP_VehicleStandstill_Ad/1
  ESP_CDD_Active_APAcv/1 -> ESP_CDD_Active_APA_F/1
  ESP_CDD_Active_APA_S/1 -> ESP_CDD_Active_APAcv/1
  ESP_CDD_Active_APA_L/1 -> ESP_CDD_Active_APA_S/1
  ESP_CDD_Active_APA_Convert/1 -> ESP_CDD_Active_APA_L/1
  ESP_CDD_Active_APA_Sub/1(Out1) -> ESP_CDD_Active_APA_Convert/1
  ESP_CDD_Active_APA_sat/1 -> ESP_CDD_Active_APA_Out/1
  ESP_CDD_Active_APA_Ad/1 -> ESP_CDD_Active_APA_sat/1
  ESP_CDD_Active_APA_O/1 -> ESP_CDD_Active_APA_Ad/2
  ESP_CDD_Active_APA_F/1 -> ESP_CDD_Active_APA_Ad/1
  ESP_CDD_Availablecv/1 -> ESP_CDD_Available_F/1
  ESP_CDD_Available_S/1 -> ESP_CDD_Availablecv/1
  ESP_CDD_Available_L/1 -> ESP_CDD_Available_S/1
  ESP_CDD_Available_Convert/1 -> ESP_CDD_Available_L/1
  ESP_CDD_Available_Sub/1(Out1) -> ESP_CDD_Available_Convert/1
  ESP_CDD_Available_sat/1 -> ESP_CDD_Available_Out/1
  ESP_CDD_Available_Ad/1 -> ESP_CDD_Available_sat/1
  ESP_CDD_Available_O/1 -> ESP_CDD_Available_Ad/2
  ESP_CDD_Available_F/1 -> ESP_CDD_Available_Ad/1
  ESP_CDD_Activecv/1 -> ESP_CDD_Active_F/1
  ESP_CDD_Active_S/1 -> ESP_CDD_Activecv/1
  ESP_CDD_Active_L/1 -> ESP_CDD_Active_S/1
  ESP_CDD_Active_Convert/1 -> ESP_CDD_Active_L/1
  ESP_CDD_Active_Sub/1(Out1) -> ESP_CDD_Active_Convert/1
  ESP_CDD_Active_sat/1 -> ESP_CDD_Active_Out/1
  ESP_CDD_Active_Ad/1 -> ESP_CDD_Active_sat/1
  ESP_CDD_Active_O/1 -> ESP_CDD_Active_Ad/2
  ESP_CDD_Active_F/1 -> ESP_CDD_Active_Ad/1
  ESP_BrakeOverHeatcv/1 -> ESP_BrakeOverHeat_F/1
  ESP_BrakeOverHeat_S/1 -> ESP_BrakeOverHeatcv/1
  ESP_BrakeOverHeat_L/1 -> ESP_BrakeOverHeat_S/1
  ESP_BrakeOverHeat_Convert/1 -> ESP_BrakeOverHeat_L/1
  ESP_BrakeOverHeat_Sub/1(Out1) -> ESP_BrakeOverHeat_Convert/1
  Demux/4 -> ESP_CDD_Available_APA_Sub/1(In1), ESP_VehicleStandstill_Sub/1(In1), ESP_CDD_Active_APA_Sub/1(In1), ESP_CDD_Available_Sub/1(In1), ESP_CDD_Active_Sub/1(In1), ESP_BrakeOverHeat_Sub/1(In1)
  ESP_BrakeOverHeat_sat/1 -> ESP_BrakeOverHeat_Out/1
  ESP_BrakeOverHeat_Ad/1 -> ESP_BrakeOverHeat_sat/1
  ESP_BrakeOverHeat_O/1 -> ESP_BrakeOverHeat_Ad/2
  ESP_BrakeOverHeat_F/1 -> ESP_BrakeOverHeat_Ad/1
  ESP_PrefillActivecv/1 -> ESP_PrefillActive_F/1
  ESP_PrefillActive_S/1 -> ESP_PrefillActivecv/1
  ESP_PrefillActive_L/1 -> ESP_PrefillActive_S/1
  ESP_PrefillActive_Convert/1 -> ESP_PrefillActive_L/1
  ESP_PrefillActive_Sub/1(Out1) -> ESP_PrefillActive_Convert/1
  ESP_PrefillActive_sat/1 -> ESP_PrefillActive_Out/1
  ESP_PrefillActive_Ad/1 -> ESP_PrefillActive_sat/1
  ESP_PrefillActive_O/1 -> ESP_PrefillActive_Ad/2
  ESP_PrefillActive_F/1 -> ESP_PrefillActive_Ad/1
  ESP_PrefillAvailablecv/1 -> ESP_PrefillAvailable_F/1
  ESP_PrefillAvailable_S/1 -> ESP_PrefillAvailablecv/1
  ESP_PrefillAvailable_L/1 -> ESP_PrefillAvailable_S/1
  ESP_PrefillAvailable_Convert/1 -> ESP_PrefillAvailable_L/1
  ESP_PrefillAvailable_Sub/1(Out1) -> ESP_PrefillAvailable_Convert/1
  ESP_PrefillAvailable_sat/1 -> ESP_PrefillAvailable_Out/1
  ESP_PrefillAvailable_Ad/1 -> ESP_PrefillAvailable_sat/1
  ESP_PrefillAvailable_O/1 -> ESP_PrefillAvailable_Ad/2
  ESP_PrefillAvailable_F/1 -> ESP_PrefillAvailable_Ad/1
  ESP_ABAactivecv/1 -> ESP_ABAactive_F/1
  ESP_ABAactive_S/1 -> ESP_ABAactivecv/1
  ESP_ABAactive_L/1 -> ESP_ABAactive_S/1
  ESP_ABAactive_Convert/1 -> ESP_ABAactive_L/1
  ESP_ABAactive_Sub/1(Out1) -> ESP_ABAactive_Convert/1
  ESP_ABAactive_sat/1 -> ESP_ABAactive_Out/1
  ESP_ABAactive_Ad/1 -> ESP_ABAactive_sat/1
  ESP_ABAactive_O/1 -> ESP_ABAactive_Ad/2
  ESP_ABAactive_F/1 -> ESP_ABAactive_Ad/1
  ESP_ABAavailablecv/1 -> ESP_ABAavailable_F/1
  ESP_ABAavailable_S/1 -> ESP_ABAavailablecv/1
  ESP_ABAavailable_L/1 -> ESP_ABAavailable_S/1
  ESP_ABAavailable_Convert/1 -> ESP_ABAavailable_L/1
  ESP_ABAavailable_Sub/1(Out1) -> ESP_ABAavailable_Convert/1
  ESP_ABAavailable_sat/1 -> ESP_ABAavailable_Out/1
  ESP_ABAavailable_Ad/1 -> ESP_ABAavailable_sat/1
  ESP_ABAavailable_O/1 -> ESP_ABAavailable_Ad/2
  ESP_ABAavailable_F/1 -> ESP_ABAavailable_Ad/1
  ESP_AEBAvailablecv/1 -> ESP_AEBAvailable_F/1
  ESP_AEBAvailable_S/1 -> ESP_AEBAvailablecv/1
  ESP_AEBAvailable_L/1 -> ESP_AEBAvailable_S/1
  ESP_AEBAvailable_Convert/1 -> ESP_AEBAvailable_L/1
  ESP_AEBAvailable_Sub/1(Out1) -> ESP_AEBAvailable_Convert/1
  ESP_AEBAvailable_sat/1 -> ESP_AEBAvailable_Out/1
  ESP_AEBAvailable_Ad/1 -> ESP_AEBAvailable_sat/1
  ESP_AEBAvailable_O/1 -> ESP_AEBAvailable_Ad/2
  ESP_AEBAvailable_F/1 -> ESP_AEBAvailable_Ad/1
  ESP_AEBdecActivecv/1 -> ESP_AEBdecActive_F/1
  ESP_AEBdecActive_S/1 -> ESP_AEBdecActivecv/1
  ESP_AEBdecActive_L/1 -> ESP_AEBdecActive_S/1
  ESP_AEBdecActive_Convert/1 -> ESP_AEBdecActive_L/1
  ESP_AEBdecActive_Sub/1(Out1) -> ESP_AEBdecActive_Convert/1
  ESP_AEBdecActive_sat/1 -> ESP_AEBdecActive_Out/1
  ESP_AEBdecActive_Ad/1 -> ESP_AEBdecActive_sat/1
  ESP_AEBdecActive_O/1 -> ESP_AEBdecActive_Ad/2
  ESP_AEBdecActive_F/1 -> ESP_AEBdecActive_Ad/1
  ESP_AWBactivecv/1 -> ESP_AWBactive_F/1
  ESP_AWBactive_S/1 -> ESP_AWBactivecv/1
  ESP_AWBactive_L/1 -> ESP_AWBactive_S/1
  ESP_AWBactive_Convert/1 -> ESP_AWBactive_L/1
  ESP_AWBactive_Sub/1(Out1) -> ESP_AWBactive_Convert/1
  ESP_AWBactive_sat/1 -> ESP_AWBactive_Out/1
  ESP_AWBactive_Ad/1 -> ESP_AWBactive_sat/1
  ESP_AWBactive_O/1 -> ESP_AWBactive_Ad/2
  ESP_AWBactive_F/1 -> ESP_AWBactive_Ad/1
  ESP_AWBavailablecv/1 -> ESP_AWBavailable_F/1
  ESP_AWBavailable_S/1 -> ESP_AWBavailablecv/1
  ESP_AWBavailable_L/1 -> ESP_AWBavailable_S/1
  ESP_AWBavailable_Convert/1 -> ESP_AWBavailable_L/1
  ESP_AWBavailable_Sub/1(Out1) -> ESP_AWBavailable_Convert/1
  Demux/3 -> ESP_PrefillActive_Sub/1(In1), ESP_PrefillAvailable_Sub/1(In1), ESP_ABAactive_Sub/1(In1), ESP_ABAavailable_Sub/1(In1), ESP_AEBAvailable_Sub/1(In1), ESP_AEBdecActive_Sub/1(In1), ESP_AWBactive_Sub/1(In1), ESP_AWBavailable_Sub/1(In1)
  ESP_AWBavailable_sat/1 -> ESP_AWBavailable_Out/1
  ESP_AWBavailable_Ad/1 -> ESP_AWBavailable_sat/1
  ESP_AWBavailable_O/1 -> ESP_AWBavailable_Ad/2
  ESP_AWBavailable_F/1 -> ESP_AWBavailable_Ad/1
  ESP_TCSActivecv/1 -> ESP_TCSActive_F/1
  ESP_TCSActive_S/1 -> ESP_TCSActivecv/1
  ESP_TCSActive_L/1 -> ESP_TCSActive_S/1
  ESP_TCSActive_Convert/1 -> ESP_TCSActive_L/1
  ESP_TCSActive_Sub/1(Out1) -> ESP_TCSActive_Convert/1
  ESP_TCSActive_sat/1 -> ESP_TCSActive_Out/1
  ESP_TCSActive_Ad/1 -> ESP_TCSActive_sat/1
  ESP_TCSActive_O/1 -> ESP_TCSActive_Ad/2
  ESP_TCSActive_F/1 -> ESP_TCSActive_Ad/1
  ESP_VDCActivecv/1 -> ESP_VDCActive_F/1
  ESP_VDCActive_S/1 -> ESP_VDCActivecv/1
  ESP_VDCActive_L/1 -> ESP_VDCActive_S/1
  ESP_VDCActive_Convert/1 -> ESP_VDCActive_L/1
  ESP_VDCActive_Sub/1(Out1) -> ESP_VDCActive_Convert/1
  ESP_VDCActive_sat/1 -> ESP_VDCActive_Out/1
  ESP_VDCActive_Ad/1 -> ESP_VDCActive_sat/1
  ESP_VDCActive_O/1 -> ESP_VDCActive_Ad/2
  ESP_VDCActive_F/1 -> ESP_VDCActive_Ad/1
  ESP_BrakeForcecv/1 -> ESP_BrakeForce_F/1
  ESP_BrakeForce_S/1 -> ESP_BrakeForcecv/1
  ESP_BrakeForce_L/1 -> ESP_BrakeForce_S/1
  ESP_BrakeForce_Convert/1 -> ESP_BrakeForce_L/1
  ESP_BrakeForce_Sub/1(Out1) -> ESP_BrakeForce_Convert/1
  Demux/2 -> ESP_TCSActive_Sub/1(In1), ESP_VDCActive_Sub/1(In1), ESP_BrakeForce_Sub/1(In1)
  ESP_BrakeForce_sat/1 -> ESP_BrakeForce_Out/1
  ESP_BrakeForce_Ad/1 -> ESP_BrakeForce_sat/1
  ESP_BrakeForce_O/1 -> ESP_BrakeForce_Ad/2
  ESP_BrakeForce_F/1 -> ESP_BrakeForce_Ad/1
